simulink model "type2_STC"  (R2024b)
settings: Solver=VariableStepAuto  StartTime=0.0  StopTime=10.0  RelTol=1e-3
libraries: simulink x3
(part 1 of 2)
settings Model: Creator=chall  LastModifiedBy=chall

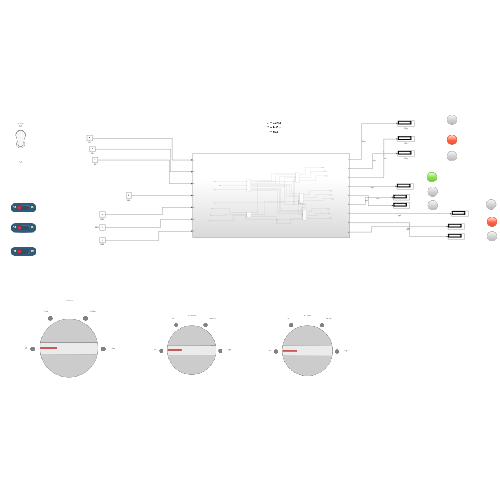
[thumbnail: Simulink's stored preview of the top-level diagram]
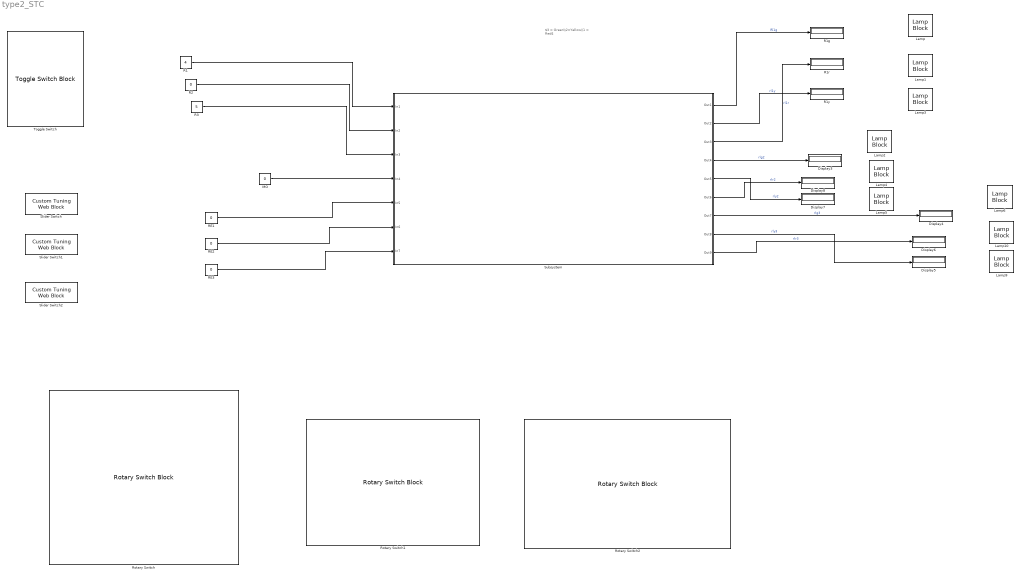
== system type2_STC ==
  note: $3 = Green\\2=Yellow\\1 = Red$
  Display{3..8} (6 alike) : Display
  Lamp{,1..6,9..10} (9 alike) : LampBlock  LabelPosition=Hide
  MO : Constant  Value=0
  R1 : Constant  Value=4
  R1g : Display
  R1r : Display
  R1y : Display
  R2 : Constant  Value=0
  R3 : Constant  Value=5
  RE1 : Constant  Value=0
  RE2 : Constant  Value=0
  RE3 : Constant  Value=0
  Rotary Switch : RotarySwitchBlock
      settings: Values={{'Off', 'Low', 'Medium', 'High'}, [0 1 2 3]}
  Rotary Switch1 : RotarySwitchBlock
      settings: Values={{'Off', 'Low', 'Medium', 'High'}, [0 1 2 3]}
  Rotary Switch2 : RotarySwitchBlock
      settings: Values={{'Off', 'Low', 'Medium', 'High'}, [0 1 2 3]}
  Slider Switch : CustomTuningWebBlock  LabelPosition=Hide  ShowInitialText=on  Configuration="{\"components\":[{\"name\":\"CustomSwitchStateComponent\",\"settings\":{\"position\":[0,0,1,1],\"states\":[{\"HitRegion\":{\"position\":[0,0,0.5,1]},\"Image\":{\"position\":[0,0,1,1],\"size\":[1,1],\"src\":\"data:image\\/svg+xml;base64,PD94bWwgdmVyc2lvbj0iMS4wIiBlbmNvZGluZz0idXRmLTgiPz4NCjwhLS0gR2VuZXJhdG9yOiBBZG9iZSBJbGx1c3RyYXRvciAyNS4yLjEsIFNWRyBFeHBvcnQgUGx1Zy1JbiAuIFNWRyBWZXJzaW9uOiA2LjAwIEJ1aWxkIDApICAtLT4NCjxzdmcgdmVyc2lvbj0iMS4xIiB4bWxucz0iaHR0cDovL3d3dy53My5vcmcvMjAwMC9zdmciIHhtbG5zOnhsaW5rPSJodHRwOi8vd3d3LnczLm9yZy8xOTk5L3hsaW5rIiB4PSIwcHgiIHk9IjBweCINCgkgdmlld0JveD0iMCAwIDc2IDI5IiBzdHlsZT0iZW5hYmxlLWJhY2tncm91bmQ6bmV3 ...(+5404 chars)\",\"srcOrientation\":\"Right\"},\"Label\":{\"color\":[0.9882352941176471,0.9882352941176471,0.7725490196078432],\"icon\":{\"size\":[0,0],\"src\":[],\"srcOrientation\":\"Right\"},\"iconPlacement\":\"left\",\"opacity\":1,\"position\":[0.5,0.14],\"show\":true,\"text\":{\"content\":\"Off\",\"font\":\"Helvetica\"}},\"Value\":0},{\"HitRegion\":{\"position\":[0,0.5,0.5,1]},\"Image\":{\"position\":[0,0,1,1],\"size\":[1,1],\"src\":\"data:image\\/svg+xml;base64,PD94bWwgdmVyc2lvbj0iMS4wIiBlbmNvZGluZz0idXRmLTgiPz4NCjwhLS0gR2VuZXJhdG9yOiBBZG9iZSBJbGx1c3RyYXRvciAyNS4yLjEsIFNWRyBFeHBvcnQgUGx1Zy1JbiAuIFNWRyBWZXJzaW9uOiA2LjAwIEJ1aWxkIDApICAtLT4NCjxzdmcgdmVyc2lvbj0iMS4xIiB4bWxucz0iaHR0cDovL3d3dy53My5vcmcvMjAwMC9zdmciIHhtbG5zOnhsaW5rPSJodHRwOi8vd3d3LnczLm9yZy8xOTk5L3hsaW5rIiB4PSIwcHgiIHk9IjBweCINCgkgdmlld0JveD0iMCAwIDc2IDI5IiBzdHlsZT0iZW5hYmxlLWJhY2tncm91bmQ6bmV3 ...(+5404 chars)\",\"srcOrientation\":\"Right\"},\"Label\":{\"color\":[0.9882352941176471,0.9882352941176471,0.7725490196078432],\"icon\":{\"size\":[0,0],\"src\":[],\"srcOrientation\":\"Right\"},\"iconPlacement\":\"left\",\"opacity\":1,\"position\":[0.5,0.86],\"show\":true,\"text\":{\"content\":\"On\",\"font\":\"Helvetica\"}},\"Value\":1}]}},{\"name\":\"BackgroundImageComponent\",\"settings\":{\"image\":{\"size\":[140,55],\"src\":\"default\",\"srcOrientation\":\"Right\"},\"position\":[0,0,1,1],\"scaleMode\":\"0\"}},{\"name\":\"ForegroundImageComponent\",\"settings\":{\"image\":{\"size\":[0,0],\"src\":\"default\",\"srcOrientation\":[]},\"isForeground\":1,\"position\":[0,0,1,1],\"scaleMode\":\"0\"}}],\"settings\":{\"BindingType\":\"param\",\"backgroundColor\":[0,0,255,\"1\"],\"backgroundOffset\":0.14,\"fixedAspectRatio\":\"on\",\"foregroundColor\":[234,234,234],\"showBackgroundColor\":false,\"variant\":\"slider\",\"version\":\"R2024b\"},\"type\":\"Switch\"}"
  Slider Switch1 : CustomTuningWebBlock  LabelPosition=Hide  ShowInitialText=on  Configuration="{\"components\":[{\"name\":\"CustomSwitchStateComponent\",\"settings\":{\"position\":[0,0,1,1],\"states\":[{\"HitRegion\":{\"position\":[0,0,0.5,1]},\"Image\":{\"position\":[0,0,1,1],\"size\":[1,1],\"src\":\"data:image\\/svg+xml;base64,PD94bWwgdmVyc2lvbj0iMS4wIiBlbmNvZGluZz0idXRmLTgiPz4NCjwhLS0gR2VuZXJhdG9yOiBBZG9iZSBJbGx1c3RyYXRvciAyNS4yLjEsIFNWRyBFeHBvcnQgUGx1Zy1JbiAuIFNWRyBWZXJzaW9uOiA2LjAwIEJ1aWxkIDApICAtLT4NCjxzdmcgdmVyc2lvbj0iMS4xIiB4bWxucz0iaHR0cDovL3d3dy53My5vcmcvMjAwMC9zdmciIHhtbG5zOnhsaW5rPSJodHRwOi8vd3d3LnczLm9yZy8xOTk5L3hsaW5rIiB4PSIwcHgiIHk9IjBweCINCgkgdmlld0JveD0iMCAwIDc2IDI5IiBzdHlsZT0iZW5hYmxlLWJhY2tncm91bmQ6bmV3 ...(+5404 chars)\",\"srcOrientation\":\"Right\"},\"Label\":{\"color\":[0.9882352941176471,0.9882352941176471,0.7725490196078432],\"icon\":{\"size\":[0,0],\"src\":[],\"srcOrientation\":\"Right\"},\"iconPlacement\":\"left\",\"opacity\":1,\"position\":[0.5,0.14],\"show\":true,\"text\":{\"content\":\"Off\",\"font\":\"Helvetica\"}},\"Value\":0},{\"HitRegion\":{\"position\":[0,0.5,0.5,1]},\"Image\":{\"position\":[0,0,1,1],\"size\":[1,1],\"src\":\"data:image\\/svg+xml;base64,PD94bWwgdmVyc2lvbj0iMS4wIiBlbmNvZGluZz0idXRmLTgiPz4NCjwhLS0gR2VuZXJhdG9yOiBBZG9iZSBJbGx1c3RyYXRvciAyNS4yLjEsIFNWRyBFeHBvcnQgUGx1Zy1JbiAuIFNWRyBWZXJzaW9uOiA2LjAwIEJ1aWxkIDApICAtLT4NCjxzdmcgdmVyc2lvbj0iMS4xIiB4bWxucz0iaHR0cDovL3d3dy53My5vcmcvMjAwMC9zdmciIHhtbG5zOnhsaW5rPSJodHRwOi8vd3d3LnczLm9yZy8xOTk5L3hsaW5rIiB4PSIwcHgiIHk9IjBweCINCgkgdmlld0JveD0iMCAwIDc2IDI5IiBzdHlsZT0iZW5hYmxlLWJhY2tncm91bmQ6bmV3 ...(+5404 chars)\",\"srcOrientation\":\"Right\"},\"Label\":{\"color\":[0.9882352941176471,0.9882352941176471,0.7725490196078432],\"icon\":{\"size\":[0,0],\"src\":[],\"srcOrientation\":\"Right\"},\"iconPlacement\":\"left\",\"opacity\":1,\"position\":[0.5,0.86],\"show\":true,\"text\":{\"content\":\"On\",\"font\":\"Helvetica\"}},\"Value\":1}]}},{\"name\":\"BackgroundImageComponent\",\"settings\":{\"image\":{\"size\":[140,55],\"src\":\"default\",\"srcOrientation\":\"Right\"},\"position\":[0,0,1,1],\"scaleMode\":\"0\"}},{\"name\":\"ForegroundImageComponent\",\"settings\":{\"image\":{\"size\":[0,0],\"src\":\"default\",\"srcOrientation\":[]},\"isForeground\":1,\"position\":[0,0,1,1],\"scaleMode\":\"0\"}}],\"settings\":{\"BindingType\":\"param\",\"backgroundColor\":[0,0,255,\"1\"],\"backgroundOffset\":0.14,\"fixedAspectRatio\":\"on\",\"foregroundColor\":[234,234,234],\"showBackgroundColor\":false,\"variant\":\"slider\",\"version\":\"R2024b\"},\"type\":\"Switch\"}"
  Slider Switch2 : CustomTuningWebBlock  LabelPosition=Hide  ShowInitialText=on  Configuration="{\"components\":[{\"name\":\"CustomSwitchStateComponent\",\"settings\":{\"position\":[0,0,1,1],\"states\":[{\"HitRegion\":{\"position\":[0,0,0.5,1]},\"Image\":{\"position\":[0,0,1,1],\"size\":[1,1],\"src\":\"data:image\\/svg+xml;base64,PD94bWwgdmVyc2lvbj0iMS4wIiBlbmNvZGluZz0idXRmLTgiPz4NCjwhLS0gR2VuZXJhdG9yOiBBZG9iZSBJbGx1c3RyYXRvciAyNS4yLjEsIFNWRyBFeHBvcnQgUGx1Zy1JbiAuIFNWRyBWZXJzaW9uOiA2LjAwIEJ1aWxkIDApICAtLT4NCjxzdmcgdmVyc2lvbj0iMS4xIiB4bWxucz0iaHR0cDovL3d3dy53My5vcmcvMjAwMC9zdmciIHhtbG5zOnhsaW5rPSJodHRwOi8vd3d3LnczLm9yZy8xOTk5L3hsaW5rIiB4PSIwcHgiIHk9IjBweCINCgkgdmlld0JveD0iMCAwIDc2IDI5IiBzdHlsZT0iZW5hYmxlLWJhY2tncm91bmQ6bmV3 ...(+5404 chars)\",\"srcOrientation\":\"Right\"},\"Label\":{\"color\":[0.9882352941176471,0.9882352941176471,0.7725490196078432],\"icon\":{\"size\":[0,0],\"src\":[],\"srcOrientation\":\"Right\"},\"iconPlacement\":\"left\",\"opacity\":1,\"position\":[0.5,0.14],\"show\":true,\"text\":{\"content\":\"Off\",\"font\":\"Helvetica\"}},\"Value\":0},{\"HitRegion\":{\"position\":[0,0.5,0.5,1]},\"Image\":{\"position\":[0,0,1,1],\"size\":[1,1],\"src\":\"data:image\\/svg+xml;base64,PD94bWwgdmVyc2lvbj0iMS4wIiBlbmNvZGluZz0idXRmLTgiPz4NCjwhLS0gR2VuZXJhdG9yOiBBZG9iZSBJbGx1c3RyYXRvciAyNS4yLjEsIFNWRyBFeHBvcnQgUGx1Zy1JbiAuIFNWRyBWZXJzaW9uOiA2LjAwIEJ1aWxkIDApICAtLT4NCjxzdmcgdmVyc2lvbj0iMS4xIiB4bWxucz0iaHR0cDovL3d3dy53My5vcmcvMjAwMC9zdmciIHhtbG5zOnhsaW5rPSJodHRwOi8vd3d3LnczLm9yZy8xOTk5L3hsaW5rIiB4PSIwcHgiIHk9IjBweCINCgkgdmlld0JveD0iMCAwIDc2IDI5IiBzdHlsZT0iZW5hYmxlLWJhY2tncm91bmQ6bmV3 ...(+5404 chars)\",\"srcOrientation\":\"Right\"},\"Label\":{\"color\":[0.9882352941176471,0.9882352941176471,0.7725490196078432],\"icon\":{\"size\":[0,0],\"src\":[],\"srcOrientation\":\"Right\"},\"iconPlacement\":\"left\",\"opacity\":1,\"position\":[0.5,0.86],\"show\":true,\"text\":{\"content\":\"On\",\"font\":\"Helvetica\"}},\"Value\":1}]}},{\"name\":\"BackgroundImageComponent\",\"settings\":{\"image\":{\"size\":[140,55],\"src\":\"default\",\"srcOrientation\":\"Right\"},\"position\":[0,0,1,1],\"scaleMode\":\"0\"}},{\"name\":\"ForegroundImageComponent\",\"settings\":{\"image\":{\"size\":[0,0],\"src\":\"default\",\"srcOrientation\":[]},\"isForeground\":1,\"position\":[0,0,1,1],\"scaleMode\":\"0\"}}],\"settings\":{\"BindingType\":\"param\",\"backgroundColor\":[0,0,255,\"1\"],\"backgroundOffset\":0.14,\"fixedAspectRatio\":\"on\",\"foregroundColor\":[234,234,234],\"showBackgroundColor\":false,\"variant\":\"slider\",\"version\":\"R2024b\"},\"type\":\"Switch\"}"
  Subsystem : Subsystem
  Toggle Switch : ToggleSwitchBlock
      settings: Values={{'Off', 'On'}, [1 0]}
  wires:
  R1/1 -> Subsystem/1(In1)
  R2/1 -> Subsystem/2(In2)
  R3/1 -> Subsystem/3(In3)
  MO/1 -> Subsystem/4(In4)
  RE1/1 -> Subsystem/5(In5)
  RE2/1 -> Subsystem/6(In6)
  RE3/1 -> Subsystem/7(In7)
  Subsystem/1(Out1) -> R1g/1  "Rl1g"
  Subsystem/2(Out2) -> R1y/1  "rl1y"
  Subsystem/3(Out3) -> R1r/1  "rl1r"
  Subsystem/4(Out4) -> Display3/1  "rlg2"
  Subsystem/5(Out5) -> Display7/1  "rly2"
  Subsystem/6(Out6) -> Display8/1  "rlr2"
  Subsystem/7(Out7) -> Display4/1  "rlg3"
  Subsystem/8(Out8) -> Display5/1  "rly3"
  Subsystem/9(Out9) -> Display6/1  "rlr3"

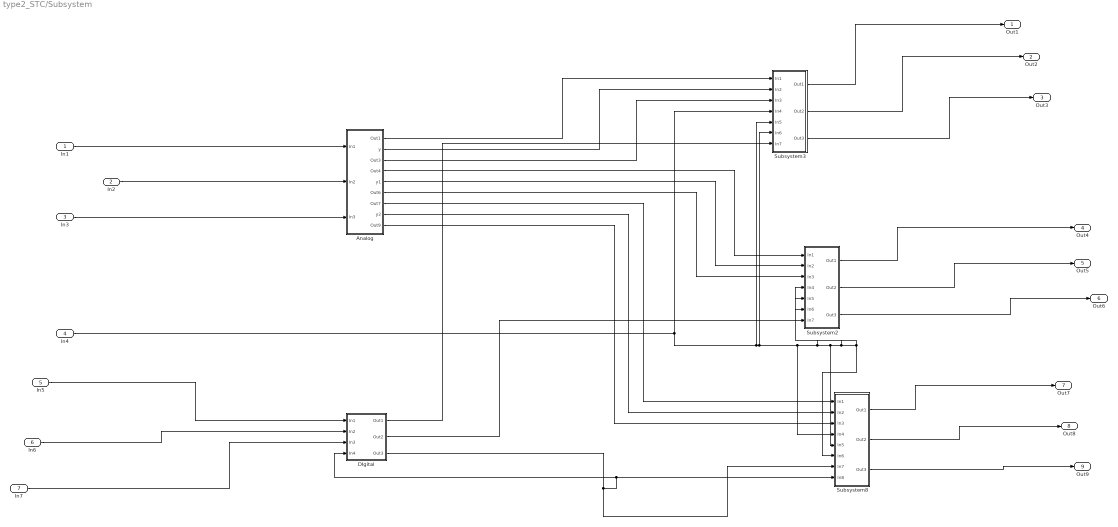
== system type2_STC/Subsystem ==
  In1 : Inport
  In2 : Inport  Port=2
  In3 : Inport  Port=3
  In4 : Inport  Port=4
  In5 : Inport  Port=5
  In6 : Inport  Port=6
  In7 : Inport  Port=7
  Analog : Subsystem
  DIgital : Subsystem
  Subsystem2 : Subsystem
  Subsystem3 : Subsystem
  Subsystem8 : Subsystem
  Out1 : Outport
  Out2 : Outport  Port=2
  Out3 : Outport  Port=3
  Out4 : Outport  Port=4
  Out5 : Outport  Port=5
  Out6 : Outport  Port=6
  Out7 : Outport  Port=7
  Out8 : Outport  Port=8
  Out9 : Outport  Port=9
  wires:
  Subsystem3/3(Out3) -> Out3/1
  Analog/2(y) -> Subsystem3/2(In2)
  In4/1 -> Subsystem3/5(In5), Subsystem8/4(In4), Subsystem2/4(In4), Subsystem8/5(In5), Subsystem2/5(In5), Subsystem2/6(In6), Subsystem8/6(In6), Subsystem3/6(In6), Subsystem3/4(In4)
  Analog/1(Out1) -> Subsystem3/1(In1)
  In1/1 -> Analog/1(In1)
  Analog/8(y2) -> Subsystem8/2(In2)
  In3/1 -> Analog/3(In3)
  Analog/3(Out3) -> Subsystem3/3(In3)
  Analog/7(Out7) -> Subsystem8/1(In1)
  Subsystem8/2(Out2) -> Out8/1
  DIgital/3(Out3) -> Subsystem8/7(In7), DIgital/4(In4), Subsystem8/8(In8)
  In6/1 -> DIgital/2(In2)
  Subsystem2/3(Out3) -> Out6/1
  In5/1 -> DIgital/1(In1)
  In2/1 -> Analog/2(In2)
  Analog/5(y1) -> Subsystem2/2(In2)
  In7/1 -> DIgital/3(In3)
  Analog/9(Out9) -> Subsystem8/3(In3)
  Subsystem8/1(Out1) -> Out7/1
  DIgital/1(Out1) -> Subsystem3/7(In7)
  DIgital/2(Out2) -> Subsystem2/7(In7)
  Subsystem3/2(Out2) -> Out2/1
  Analog/6(Out6) -> Subsystem2/3(In3)
  Subsystem3/1(Out1) -> Out1/1
  Analog/4(Out4) -> Subsystem2/1(In1)
  Subsystem8/3(Out3) -> Out9/1
  Subsystem2/2(Out2) -> Out5/1
  Subsystem2/1(Out1) -> Out4/1

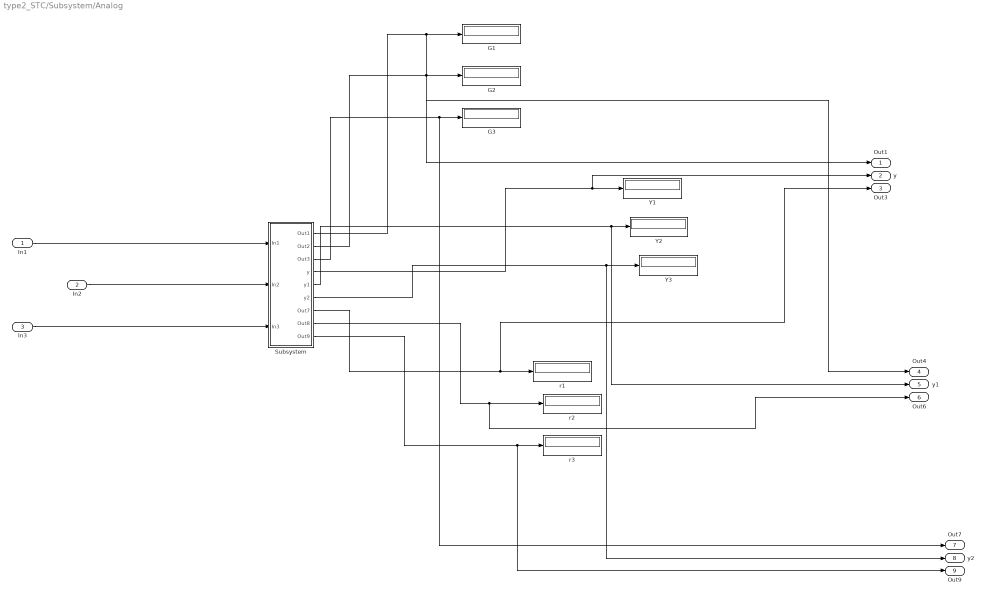
== system type2_STC/Subsystem/Analog ==
  In1 : Inport
  In2 : Inport  Port=2
  In3 : Inport  Port=3
  G1 : Display
  G2 : Display
  G3 : Display
  Subsystem : Subsystem
  Y1 : Display
  Y2 : Display
  Y3 : Display
  r1 : Display
  r2 : Display
  r3 : Display
  Out1 : Outport
  y : Outport  Port=2
  Out3 : Outport  Port=3
  Out4 : Outport  Port=4
  y1 : Outport  Port=5
  Out6 : Outport  Port=6
  Out7 : Outport  Port=7
  y2 : Outport  Port=8
  Out9 : Outport  Port=9
  wires:
  Subsystem/6(y2) -> y2/1, Y3/1
  Subsystem/4(y) -> y/1, Y1/1
  Subsystem/5(y1) -> y1/1, Y2/1
  Subsystem/3(Out3) -> Out7/1, G3/1
  Subsystem/9(Out9) -> Out9/1, r3/1
  In1/1 -> Subsystem/1(In1)
  Subsystem/1(Out1) -> Out1/1, G1/1
  Subsystem/2(Out2) -> Out4/1, G2/1
  Subsystem/8(Out8) -> Out6/1, r2/1
  Subsystem/7(Out7) -> Out3/1, r1/1
  In3/1 -> Subsystem/3(In3)
  In2/1 -> Subsystem/2(In2)

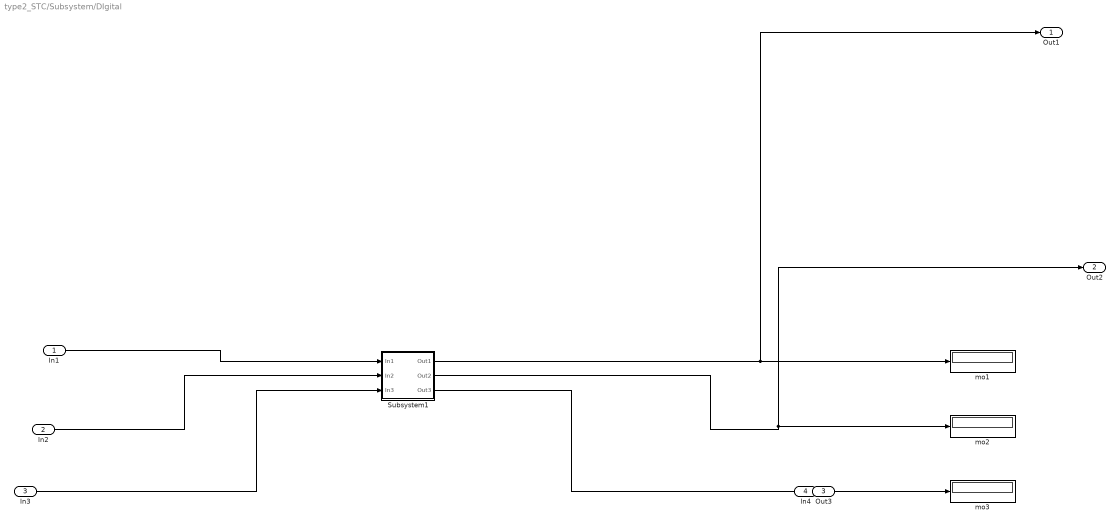
== system type2_STC/Subsystem/DIgital ==
  In1 : Inport
  In2 : Inport  Port=2
  In3 : Inport  Port=3
  In4 : Inport  Port=4
  Subsystem1 : Subsystem
  mo1 : Display
  mo2 : Display
  mo3 : Display
  Out1 : Outport
  Out2 : Outport  Port=2
  Out3 : Outport  Port=3
  wires:
  In1/1 -> Subsystem1/1(In1)
  Subsystem1/1(Out1) -> Out1/1, mo1/1
  Subsystem1/2(Out2) -> Out2/1, mo2/1
  Subsystem1/3(Out3) -> Out3/1
  In4/1 -> mo3/1
  In3/1 -> Subsystem1/3(In3)
  In2/1 -> Subsystem1/2(In2)

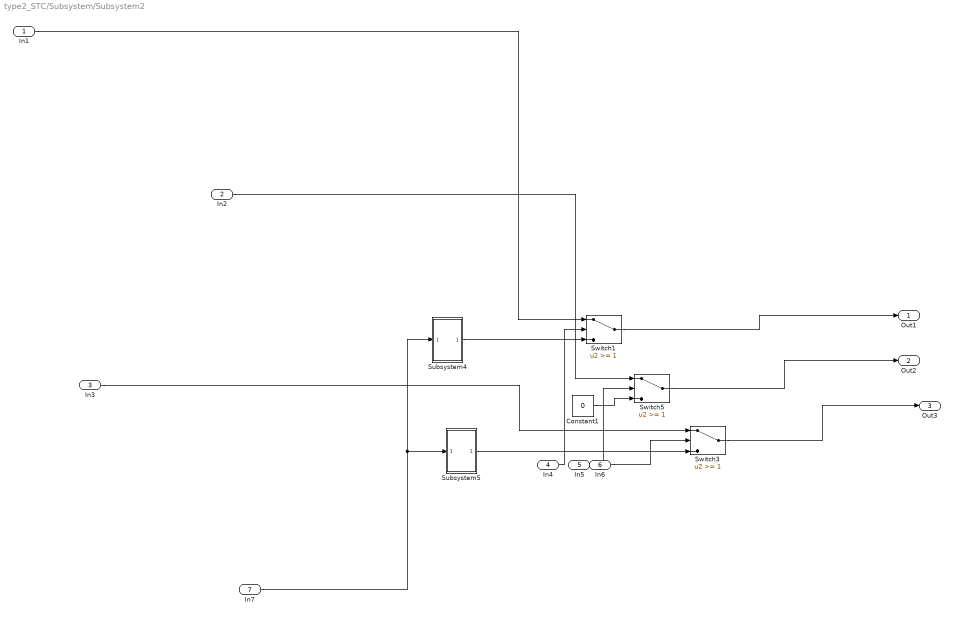
== system type2_STC/Subsystem/Subsystem2 ==
  In1 : Inport
  In2 : Inport  Port=2
  In3 : Inport  Port=3
  In4 : Inport  Port=4
  In5 : Inport  Port=5
  In6 : Inport  Port=6
  In7 : Inport  Port=7
  Constant1 : Constant  Value=0
  Subsystem4 : Subsystem
  Subsystem5 : Subsystem
  Switch1 : Switch  Threshold=1  SaturateOnIntegerOverflow=off  InputSameDT=off
  Switch3 : Switch  Threshold=1  SaturateOnIntegerOverflow=off  InputSameDT=off
  Switch5 : Switch  Threshold=1  SaturateOnIntegerOverflow=off  InputSameDT=off
  Out1 : Outport
  Out2 : Outport  Port=2
  Out3 : Outport  Port=3
  wires:
  In7/1 -> Subsystem5/1(In1), Subsystem4/1(In1)
  In3/1 -> Switch3/1
  Subsystem4/1(Out1) -> Switch1/3
  In2/1 -> Switch5/1
  Constant1/1 -> Switch5/3
  Subsystem5/1(Out1) -> Switch3/3
  Switch3/1 -> Out3/1
  In1/1 -> Switch1/1
  In6/1 -> Switch3/2
  Switch1/1 -> Out1/1
  Switch5/1 -> Out2/1
  In5/1 -> Switch5/2
  In4/1 -> Switch1/2

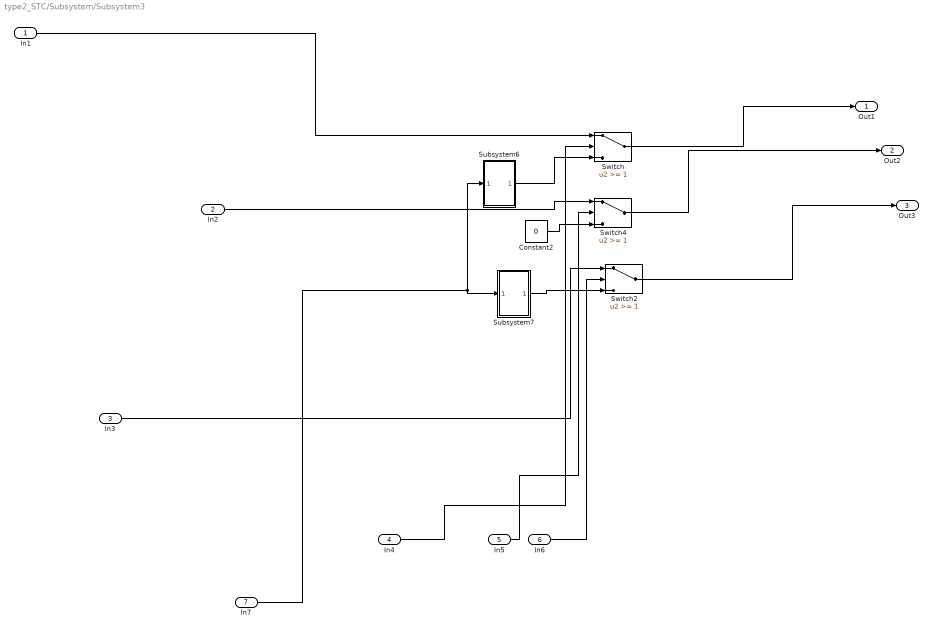
== system type2_STC/Subsystem/Subsystem3 ==
  In1 : Inport
  In2 : Inport  Port=2
  In3 : Inport  Port=3
  In4 : Inport  Port=4
  In5 : Inport  Port=5
  In6 : Inport  Port=6
  In7 : Inport  Port=7
  Constant2 : Constant  Value=0
  Subsystem6 : Subsystem
  Subsystem7 : Subsystem
  Switch : Switch  Threshold=1  SaturateOnIntegerOverflow=off  InputSameDT=off
  Switch2 : Switch  Threshold=1  SaturateOnIntegerOverflow=off  InputSameDT=off
  Switch4 : Switch  Threshold=1  SaturateOnIntegerOverflow=off  InputSameDT=off
  Out1 : Outport
  Out2 : Outport  Port=2
  Out3 : Outport  Port=3
  wires:
  In4/1 -> Switch/2
  In7/1 -> Subsystem6/1(In1), Subsystem7/1(In1)
  Constant2/1 -> Switch4/3
  Subsystem6/1(Out1) -> Switch/3
  In2/1 -> Switch4/1
  In5/1 -> Switch4/2
  Subsystem7/1(Out1) -> Switch2/3
  Switch2/1 -> Out3/1
  In3/1 -> Switch2/1
  Switch4/1 -> Out2/1
  In6/1 -> Switch2/2
  In1/1 -> Switch/1
  Switch/1 -> Out1/1

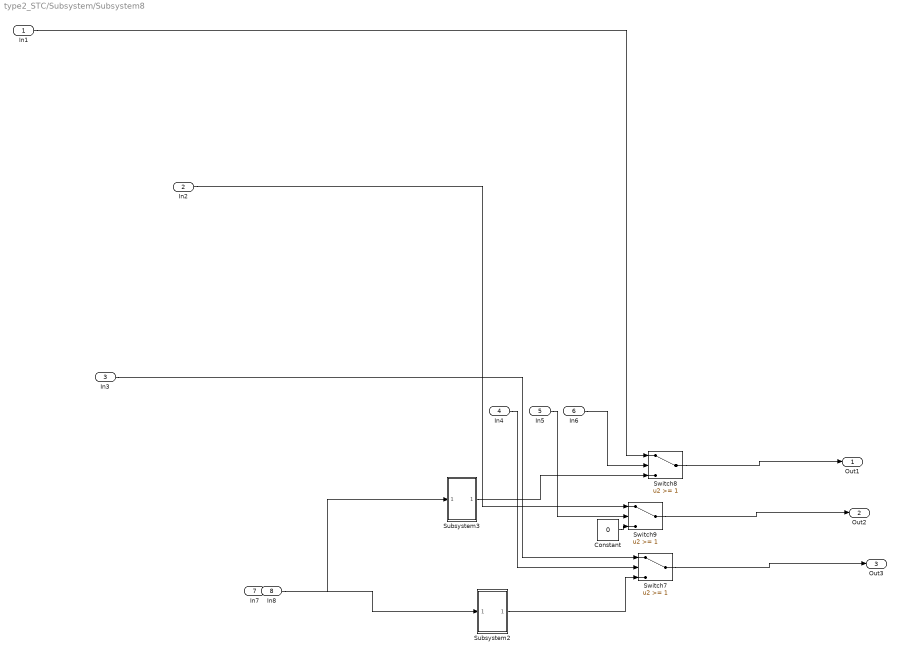
== system type2_STC/Subsystem/Subsystem8 ==
  In1 : Inport
  In2 : Inport  Port=2
  In3 : Inport  Port=3
  In4 : Inport  Port=4
  In5 : Inport  Port=5
  In6 : Inport  Port=6
  In7 : Inport  Port=7
  In8 : Inport  Port=8
  Constant : Constant  Value=0
  Subsystem2 : Subsystem
  Subsystem3 : Subsystem
  Switch7 : Switch  Threshold=1  SaturateOnIntegerOverflow=off  InputSameDT=off
  Switch8 : Switch  Threshold=1  SaturateOnIntegerOverflow=off  InputSameDT=off
  Switch9 : Switch  Threshold=1  SaturateOnIntegerOverflow=off  InputSameDT=off
  Out1 : Outport
  Out2 : Outport  Port=2
  Out3 : Outport  Port=3
  wires:
  Subsystem2/1(Out1) -> Switch7/3
  In5/1 -> Switch9/2
  In7/1 -> Subsystem2/1(In1)
  Subsystem3/1(Out1) -> Switch8/3
  Switch7/1 -> Out3/1
  In1/1 -> Switch8/1
  In8/1 -> Subsystem3/1(In1)
  Constant/1 -> Switch9/3
  In3/1 -> Switch7/1
  Switch8/1 -> Out1/1
  Switch9/1 -> Out2/1
  In6/1 -> Switch8/2
  In2/1 -> Switch9/1
  In4/1 -> Switch7/2

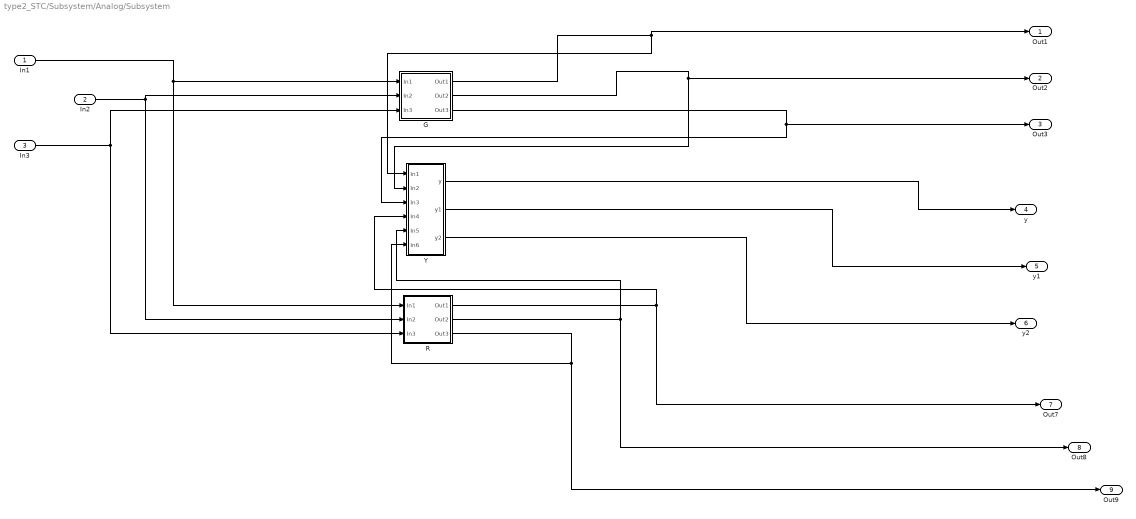
== system type2_STC/Subsystem/Analog/Subsystem ==
  In1 : Inport
  In2 : Inport  Port=2
  In3 : Inport  Port=3
  G : Subsystem
  R : Subsystem
  Y : Subsystem
  Out1 : Outport
  Out2 : Outport  Port=2
  Out3 : Outport  Port=3
  y : Outport  Port=4
  y1 : Outport  Port=5
  y2 : Outport  Port=6
  Out7 : Outport  Port=7
  Out8 : Outport  Port=8
  Out9 : Outport  Port=9
  wires:
  In3/1 -> R/3(In3), G/3(In3)
  In2/1 -> R/2(In2), G/2(In2)
  In1/1 -> R/1(In1), G/1(In1)
  G/1(Out1) -> Out1/1, Y/1(In1)
  R/2(Out2) -> Out8/1, Y/5(In5)
  G/3(Out3) -> Out3/1, Y/3(In3)
  G/2(Out2) -> Out2/1, Y/2(In2)
  R/1(Out1) -> Y/4(In4), Out7/1
  R/3(Out3) -> Out9/1, Y/6(In6)
  Y/3(y2) -> y2/1
  Y/2(y1) -> y1/1
  Y/1(y) -> y/1

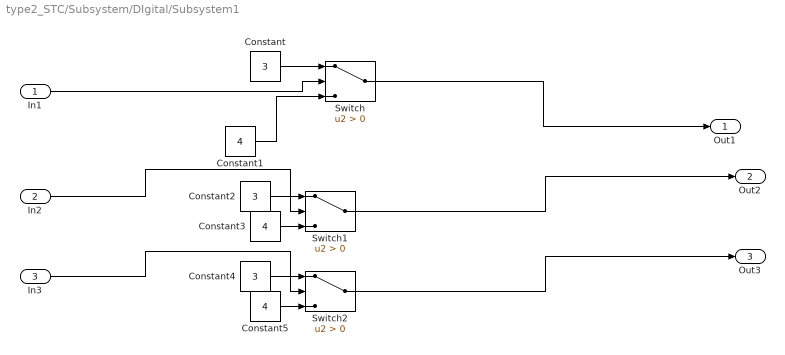
== system type2_STC/Subsystem/DIgital/Subsystem1 ==
  In1 : Inport
  In2 : Inport  Port=2
  In3 : Inport  Port=3
  Constant : Constant  Value=3
  Constant1 : Constant  Value=4
  Constant2 : Constant  Value=3
  Constant3 : Constant  Value=4
  Constant4 : Constant  Value=3
  Constant5 : Constant  Value=4
  Switch : Switch  Criteria=u2 > Threshold  SaturateOnIntegerOverflow=off  InputSameDT=off
  Switch1 : Switch  Criteria=u2 > Threshold  SaturateOnIntegerOverflow=off  InputSameDT=off
  Switch2 : Switch  Criteria=u2 > Threshold  SaturateOnIntegerOverflow=off  InputSameDT=off
  Out1 : Outport
  Out2 : Outport  Port=2
  Out3 : Outport  Port=3
  wires:
  Constant5/1 -> Switch2/3
  Constant2/1 -> Switch1/1
  Switch1/1 -> Out2/1
  Constant1/1 -> Switch/3
  Constant4/1 -> Switch2/1
  Constant/1 -> Switch/1
  Constant3/1 -> Switch1/3
  Switch2/1 -> Out3/1
  In2/1 -> Switch1/2
  In3/1 -> Switch2/2
  Switch/1 -> Out1/1
  In1/1 -> Switch/2

== system type2_STC/Subsystem/Subsystem2/Subsystem4 ==
  In1 : Inport
  Constant3 : Constant  Value=0
  Switch10 : Switch  Criteria=u2 > Threshold  Threshold=3  SaturateOnIntegerOverflow=off  InputSameDT=off
  Out1 : Outport
  wires:
  In1/1 -> Switch10/2, Switch10/3
  Constant3/1 -> Switch10/1
  Switch10/1 -> Out1/1

== system type2_STC/Subsystem/Subsystem2/Subsystem5 ==
  In1 : Inport
  Constant1 : Constant
  Constant2 : Constant  Value=0
  Switch6 : Switch  Criteria=u2 > Threshold  Threshold=3  SaturateOnIntegerOverflow=off  InputSameDT=off
  Out1 : Outport
  wires:
  Constant2/1 -> Switch6/3
  Switch6/1 -> Out1/1
  Constant1/1 -> Switch6/1
  In1/1 -> Switch6/2

== system type2_STC/Subsystem/Subsystem3/Subsystem6 ==
  In1 : Inport
  Constant3 : Constant  Value=0
  Switch10 : Switch  Criteria=u2 > Threshold  Threshold=3  SaturateOnIntegerOverflow=off  InputSameDT=off
  Out1 : Outport
  wires:
  In1/1 -> Switch10/2, Switch10/3
  Constant3/1 -> Switch10/1
  Switch10/1 -> Out1/1
